simulink model "Parallel_States"  (R2018b)
settings: Solver=FixedStepDiscrete  StartTime=0.0  StopTime=10.0  FixedStep=0.5  RelTol=1e-3
libraries: simulink x2
settings Model: Creator=marwan  LastModifiedBy=marwan

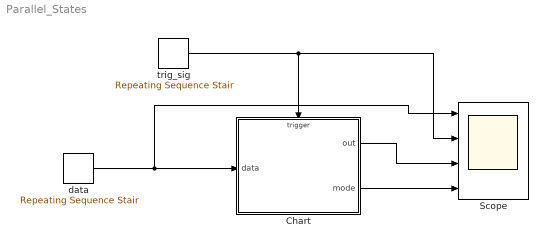
== system Parallel_States ==
  Chart : Stateflow chart  TreatAsAtomicUnit=on
  Scope : Scope  NumInputPorts=4
  data : simulink/Sources/Repeating Sequence Stair  OutValues=[0 1 2 3 4 5]  tsamp=-1  OutMin=[]  OutMax=[]  OutDataTypeStr=double  OutputDataTypeScalingMode=double  OutDataType=fixdt(0,8)  ConRadixGroup=Best Precision: Vector-wise  OutScaling=2^-12
  trig_sig : simulink/Sources/Repeating Sequence Stair  OutValues=[0 1]  tsamp=-1  OutMin=[]  OutMax=[]  OutDataTypeStr=double  OutputDataTypeScalingMode=double  OutDataType=fixdt(0,8)  ConRadixGroup=Best Precision: Vector-wise  OutScaling=2^-12
  wires:
  data/1 -> Scope/1, Chart/1(data)
  trig_sig/1 -> Chart/Trigger, Scope/2
  Chart/1(out) -> Scope/3
  Chart/2(mode) -> Scope/4

== stateflow chart Parallel_States/Chart ==
  settings: executeAtInitialization=1
  note: To make it parallel, right click here and choose Decomposition -> AND
  state State_det [parallel]
    settings: executionOrder=1
    note: decide the mode
    state on_ct
      en: i=1;
      en: mode=1;
      du: i=i+1;
    state off_ct
      en: i=1;
      en: mode=0;
      du: i=i+1;
    (default) -> on_ct
    on_ct -> off_ct : [i>=8]
    off_ct -> on_ct : [i>=2]
  state action [parallel]
    settings: executionOrder=2
    state on
      en: out=data;
      du: out=data;
    state off
      en: out=0;
      du: out=0;
    (default) -> on
    on -> off : [mode==0]
    off -> on : [mode==1]
  note: take action
  (default) -> State_det
  data: data input; out output; mode output; i local
  events: trig_sig input RISING_EDGE_EVENT
